simulink model "ARGUELLES_NO3_SIMULINK"  (R2023b)
settings: Solver=VariableStepAuto  StartTime=0.0  StopTime=20  RelTol=1e-3
values from neighbouring files (symbols this model uses):
  G_den = [b c d]    [ARGUELLES_NO3.m]    (also in ARGUELLES_NO4.m = [b c]; boo_no7.m = [f g h i j k])
  G_num = [1]    [ARGUELLES_NO3.m]    (also in ARGUELLES_NO4.m; boo_no7.m = [a b c d e])
settings Model: Creator=HP  LastModifiedBy=HP

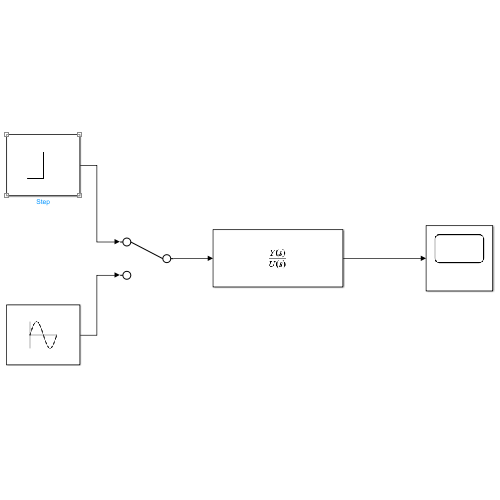
[thumbnail: Simulink's stored preview of the top-level diagram]
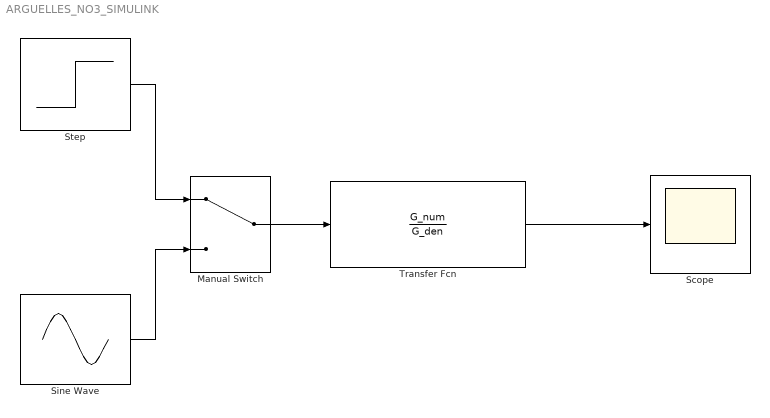
== system ARGUELLES_NO3_SIMULINK ==
  Manual Switch : ManualSwitch
  Scope : Scope
  Sine Wave : Sin  SampleTime=0
  Step : Step  Time=0  SampleTime=0
  Transfer Fcn : TransferFcn  Numerator=G_num  Denominator=G_den
  wires:
  Transfer Fcn/1 -> Scope/1
  Step/1 -> Manual Switch/1
  Manual Switch/1 -> Transfer Fcn/1
  Sine Wave/1 -> Manual Switch/2
